simulink model "LongitudinalControlLaw"  (R2020b)
settings: Solver=VariableStepAuto  StartTime=0.0  StopTime=20.0  RelTol=1e-3
undefined symbols (not defined in the file or in its folder): A, B
libraries: simulink_extras x3
settings Model: Creator=JaimeParker  LastModifiedBy=JaimeParker

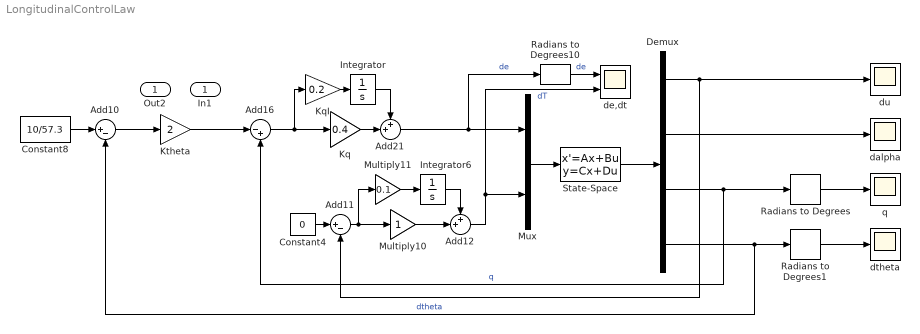
== system LongitudinalControlLaw ==
  In1 : Inport
  Add10 : Sum  Inputs=|+-
  Add11 : Sum  Inputs=|+-
  Add12 : Sum  Inputs=++|
  Add16 : Sum  Inputs=|-+
  Add21 : Sum  Inputs=++|
  Constant4 : Constant  Value=0
  Constant8 : Constant  Value=10/57.3
  Demux : Demux
  Integrator : Integrator
  Integrator6 : Integrator
  Kq : Gain  Gain=0.4
  KqI : Gain  Gain=0.2
  Ktheta : Gain  Gain=2
  Multiply10 : Gain
  Multiply11 : Gain  Gain=0.1
  Mux : Mux  Inputs=2
  Radians to Degrees : simulink_extras/Transformations/Radians to Degrees
  Radians to Degrees1 : simulink_extras/Transformations/Radians to Degrees
  Radians to Degrees10 : simulink_extras/Transformations/Radians to Degrees
  State-Space : StateSpace  A=A  B=B  C=eye(4)  D=zeros(4,2)  InitialCondition=[0;0;0;0]
  dalpha : Scope
  de,dt : Scope  NumInputPorts=2
  dtheta : Scope
  du : Scope
  q : Scope
  Out2 : Outport
  wires:
  Ktheta/1 -> Add16/1
  Kq/1 -> Add21/2
  Mux/1 -> State-Space/1
  Demux/1 -> du/1, Add11/2
  KqI/1 -> Integrator/1
  Demux/4 -> Radians to Degrees1/1, Add10/2  "dtheta"
  Multiply10/1 -> Add12/2
  Multiply11/1 -> Integrator6/1
  Integrator6/1 -> Add12/1
  Add12/1 -> Mux/2, de,dt/2  "dT"
  Demux/3 -> Radians to Degrees/1, Add16/2  "q"
  Radians to Degrees1/1 -> dtheta/1
  Constant4/1 -> Add11/1
  Integrator/1 -> Add21/1
  Add21/1 -> Radians to Degrees10/1, Mux/1  "de"
  State-Space/1 -> Demux/1
  Add11/1 -> Multiply11/1, Multiply10/1
  Demux/2 -> dalpha/1
  Radians to Degrees/1 -> q/1
  Constant8/1 -> Add10/1
  Add16/1 -> KqI/1, Kq/1
  Add10/1 -> Ktheta/1
  Radians to Degrees10/1 -> de,dt/1  "de"
